simulink model "internal_model_test"  (R2022a)
settings: Solver=VariableStepAuto  StartTime=0.0  StopTime=10  RelTol=1e-3
values from neighbouring files (symbols this model uses):
  A = zeros(6)    [find_path_coeffs.m]    (also in getLateralDynamics.m = [0 1 vx 0)
  B = [0; -b1; 0; -b2]    [getLateralDynamics.m]
  Klat = place(A, B, poles)    [lat_sim_parameters.m]    (also in tuneLateralController.m)
settings Model: Creator=fvall  LastModifiedBy=fvall

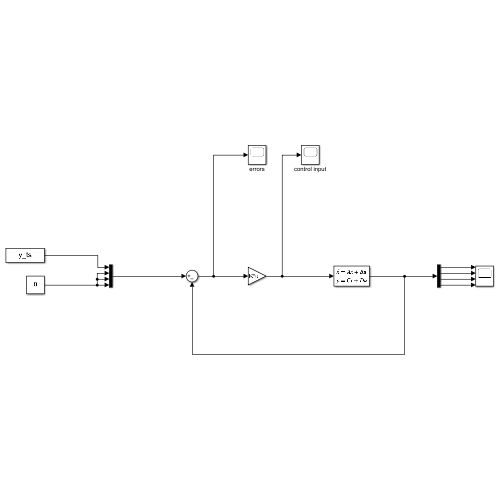
[thumbnail: Simulink's stored preview of the top-level diagram]
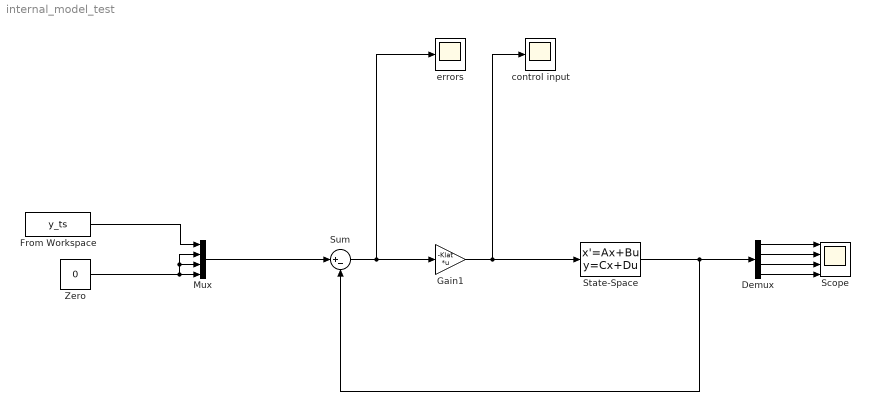
== system internal_model_test ==
  Demux : Demux
  From Workspace : FromWorkspace  VariableName=y_ts
  Gain1 : Gain  Gain=-Klat  Multiplication=Matrix(K*u)
  Mux : Mux
  Scope : Scope  NumInputPorts=4
  State-Space : StateSpace  A=A  B=B  C=eye(4)  D=zeros(4, 1)  InitialCondition=[0; 0 ; 0; 0]
  Sum : Sum  Inputs=|+-
  Zero : Constant  Value=0  OutDataTypeStr=Inherit: Inherit via back propagation
  control input : Scope
  errors : Scope
  wires:
  From Workspace/1 -> Mux/1
  Sum/1 -> Gain1/1, errors/1
  Zero/1 -> Mux/2, Mux/3, Mux/4
  Mux/1 -> Sum/1
  Gain1/1 -> State-Space/1, control input/1
  State-Space/1 -> Sum/2, Demux/1
  Demux/1 -> Scope/1
  Demux/2 -> Scope/2
  Demux/3 -> Scope/3
  Demux/4 -> Scope/4
